simulink model "F450_model"  (R2022a)
settings: Solver=ode4  StartTime=0.0  StopTime=10  FixedStep=0.001  RelTol=1e-3
values from neighbouring files (symbols this model uses):
  motorRpm0 = [5320.31451534 5320.31451534 5320.31451534 5320.31451534]    [trim_hover.mat]
  x0 = [0 0 0 0 0 0 0 0 0 0 0 -100]    [trim_hover.mat]
undefined symbols (not defined in the file or in its folder): Cd, Cmd, d_prop, dzcg, g, Inertia, Inertia_inv, Mass, motorCr, motorJm, motorTm, motorWb, rotorCm, rotorCt
libraries: matrix_library x2, aerospace x2
settings Model: SimulationMode=accelerator  Creator=dream  LastModifiedBy=김응태
settings SolverCC: AlgebraicLoopSolver=TrustRegion
settings DataIOCC: ReturnWorkspaceOutputs=off
settings DebuggingCC: UnconnectedInputMsg=warning  UnconnectedOutputMsg=warning  UnconnectedLineMsg=warning  BusObjectLabelMismatch=error  SFMachineParentedDataDiag=warning  ArithmeticOperatorsInVariantConditions=warning
settings SFSimCC: SimUseLocalCustomCode=off  CustomCodeUndefinedFunction=UseInterfaceOnly
settings RTWCC: RTWUseLocalCustomCode=off
settings CodeAppCC: StateflowObjectComments=on

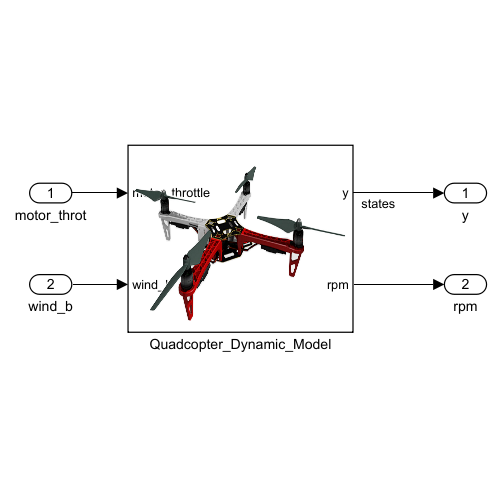
[thumbnail: Simulink's stored preview of the top-level diagram]
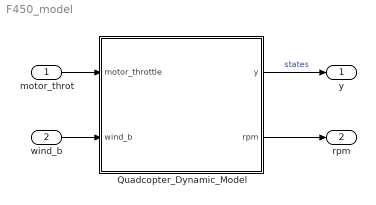
== system F450_model ==
  motor_throt : Inport
  wind_b : Inport  Port=2  PortDimensions=3
  Quadcopter_Dynamic_Model : Subsystem
      mask Display: image('F450.png'); % Use "Edit Image" on toolstrip to change.
  y : Outport
  rpm : Outport  Port=2
  wires:
  motor_throt/1 -> Quadcopter_Dynamic_Model/1(motor_throttle)
  Quadcopter_Dynamic_Model/1(y) -> y/1  "states"
  Quadcopter_Dynamic_Model/2(rpm) -> rpm/1
  wind_b/1 -> Quadcopter_Dynamic_Model/2(wind_b)

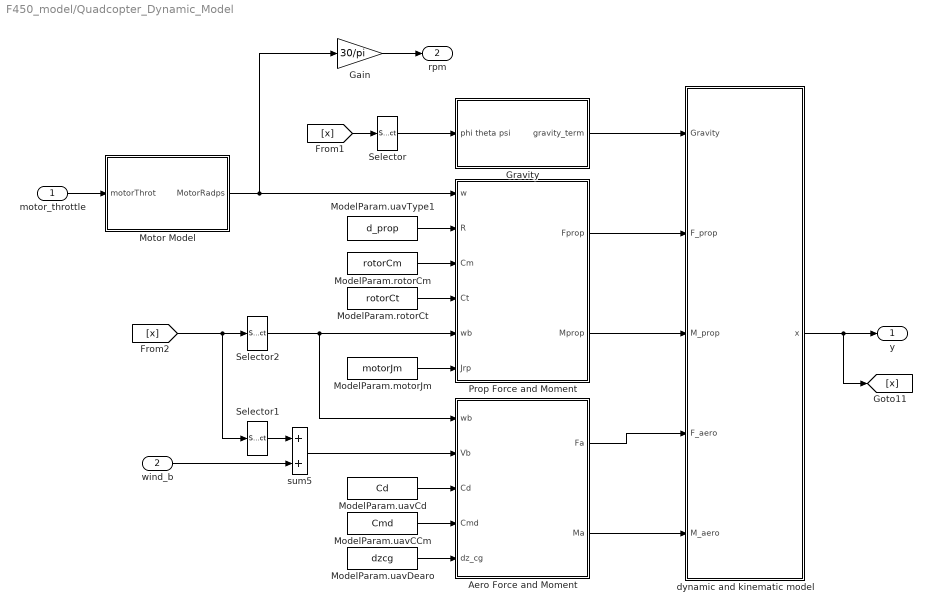
== system F450_model/Quadcopter_Dynamic_Model ==
  motor_throttle : Inport
  wind_b : Inport  Port=2
  Aero Force and Moment : MATLAB Function  TreatAsAtomicUnit=on
  Gain : Gain  Gain=30/pi
  Gravity : Subsystem
  ModelParam.motorJm : Constant  Value=motorJm
  ModelParam.rotorCm : Constant  Value=rotorCm
  ModelParam.rotorCt : Constant  Value=rotorCt
  ModelParam.uavCCm : Constant  Value=Cmd
  ModelParam.uavCd : Constant  Value=Cd
  ModelParam.uavDearo : Constant  Value=dzcg
  ModelParam.uavType1 : Constant  Value=d_prop
  Motor Model : Subsystem
  Prop Force and Moment : MATLAB Function  TreatAsAtomicUnit=on
  Selector : Selector  InputPortWidth=12  IndexOptions=Index vector (dialog)  Indices=[7 8 9]  OutputSizes=1
  Selector1 : Selector  InputPortWidth=12  IndexOptions=Index vector (dialog)  Indices=[1 2 3]  OutputSizes=1
  Selector2 : Selector  InputPortWidth=12  IndexOptions=Index vector (dialog)  Indices=[4 5 6]  OutputSizes=1
  dynamic and kinematic model : Subsystem
  sum5 : Sum  InputSameDT=on  SaturateOnIntegerOverflow=on  OutDataTypeStr=Inherit: Same as first input
  y : Outport
  rpm : Outport  Port=2
  wires:
  ModelParam.uavDearo/1 -> Aero Force and Moment/5(dz_cg)
  ModelParam.uavCCm/1 -> Aero Force and Moment/4(Cmd)
  ModelParam.uavCd/1 -> Aero Force and Moment/3(Cd)
  Aero Force and Moment/2(Ma) -> dynamic and kinematic model/5(M_aero)
  Aero Force and Moment/1(Fa) -> dynamic and kinematic model/4(F_aero)
  Prop Force and Moment/2(Mprop) -> dynamic and kinematic model/3(M_prop)
  Prop Force and Moment/1(Fprop) -> dynamic and kinematic model/2(F_prop)
  ModelParam.motorJm/1 -> Prop Force and Moment/6(Jrp)
  ModelParam.uavType1/1 -> Prop Force and Moment/2(R)
  ModelParam.rotorCt/1 -> Prop Force and Moment/4(Ct)
  ModelParam.rotorCm/1 -> Prop Force and Moment/3(Cm)
  dynamic and kinematic model/1(x) -> [x], y/1
  Gravity/1(gravity_term) -> dynamic and kinematic model/1(Gravity)
  motor_throttle/1 -> Motor Model/1(motorThrot)
  Gain/1 -> rpm/1
  Selector/1 -> Gravity/1(phi theta psi)
  [x] -> Selector/1
  [x] -> Selector2/1, Selector1/1
  Selector2/1 -> Prop Force and Moment/5(wb), Aero Force and Moment/1(wb)
  Motor Model/1(MotorRadps) -> Gain/1, Prop Force and Moment/1(w)
  wind_b/1 -> sum5/2
  Selector1/1 -> sum5/1
  sum5/1 -> Aero Force and Moment/2(Vb)

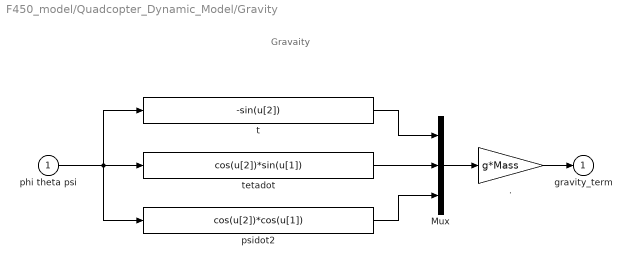
== system F450_model/Quadcopter_Dynamic_Model/Gravity ==
  note: Gravaity
  phi theta psi : Inport
  . : Gain  Gain=g*Mass  SaturateOnIntegerOverflow=on  OutDataTypeStr=Inherit: Same as input  ParamDataTypeStr=Inherit: Same as input
  Mux : Mux  Inputs=3
  psidot2 : Fcn  Expr=cos(u[2])*cos(u[1])
  t : Fcn  Expr=-sin(u[2])
  tetadot : Fcn  Expr=cos(u[2])*sin(u[1])
  gravity_term : Outport  InitialOutput=0  VectorParamsAs1DForOutWhenUnconnected=off
  wires:
  t/1 -> Mux/1
  psidot2/1 -> Mux/3
  tetadot/1 -> Mux/2
  Mux/1 -> ./1
  phi theta psi/1 -> tetadot/1, t/1, psidot2/1
  ./1 -> gravity_term/1

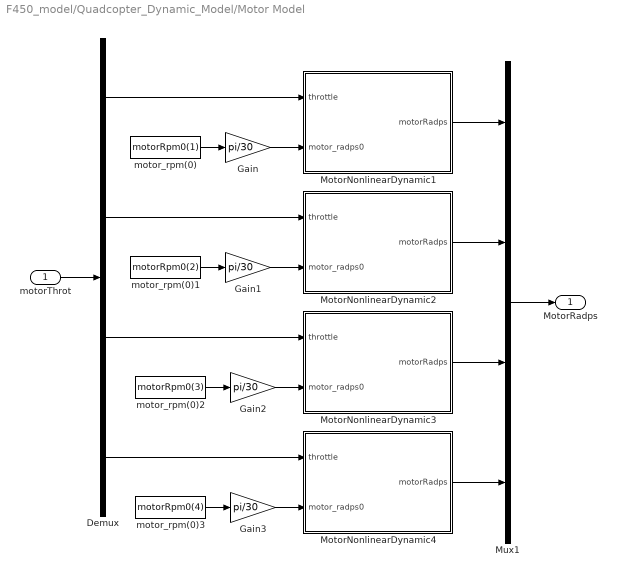
== system F450_model/Quadcopter_Dynamic_Model/Motor Model ==
  motorThrot : Inport
  Demux : Demux
  Gain{,1..3} (4 alike) : Gain  Gain=pi/30
  MotorNonlinearDynamic1 : Subsystem  TreatAsAtomicUnit=on
  MotorNonlinearDynamic2 : Subsystem  TreatAsAtomicUnit=on
  MotorNonlinearDynamic3 : Subsystem  TreatAsAtomicUnit=on
  MotorNonlinearDynamic4 : Subsystem  TreatAsAtomicUnit=on
  Mux1 : Mux
  motor_rpm(0) : Constant  Value=motorRpm0(1)
  motor_rpm(0)1 : Constant  Value=motorRpm0(2)
  motor_rpm(0)2 : Constant  Value=motorRpm0(3)
  motor_rpm(0)3 : Constant  Value=motorRpm0(4)
  MotorRadps : Outport  VectorParamsAs1DForOutWhenUnconnected=off
  wires:
  motorThrot/1 -> Demux/1
  Demux/4 -> MotorNonlinearDynamic4/1(throttle)
  motor_rpm(0)/1 -> Gain/1
  MotorNonlinearDynamic3/1(motorRadps) -> Mux1/3
  MotorNonlinearDynamic2/1(motorRadps) -> Mux1/2
  Mux1/1 -> MotorRadps/1
  Demux/2 -> MotorNonlinearDynamic2/1(throttle)
  Demux/3 -> MotorNonlinearDynamic3/1(throttle)
  Demux/1 -> MotorNonlinearDynamic1/1(throttle)
  MotorNonlinearDynamic4/1(motorRadps) -> Mux1/4
  MotorNonlinearDynamic1/1(motorRadps) -> Mux1/1
  Gain/1 -> MotorNonlinearDynamic1/2(motor_radps0)
  motor_rpm(0)1/1 -> Gain1/1
  Gain1/1 -> MotorNonlinearDynamic2/2(motor_radps0)
  motor_rpm(0)2/1 -> Gain2/1
  Gain2/1 -> MotorNonlinearDynamic3/2(motor_radps0)
  motor_rpm(0)3/1 -> Gain3/1
  Gain3/1 -> MotorNonlinearDynamic4/2(motor_radps0)

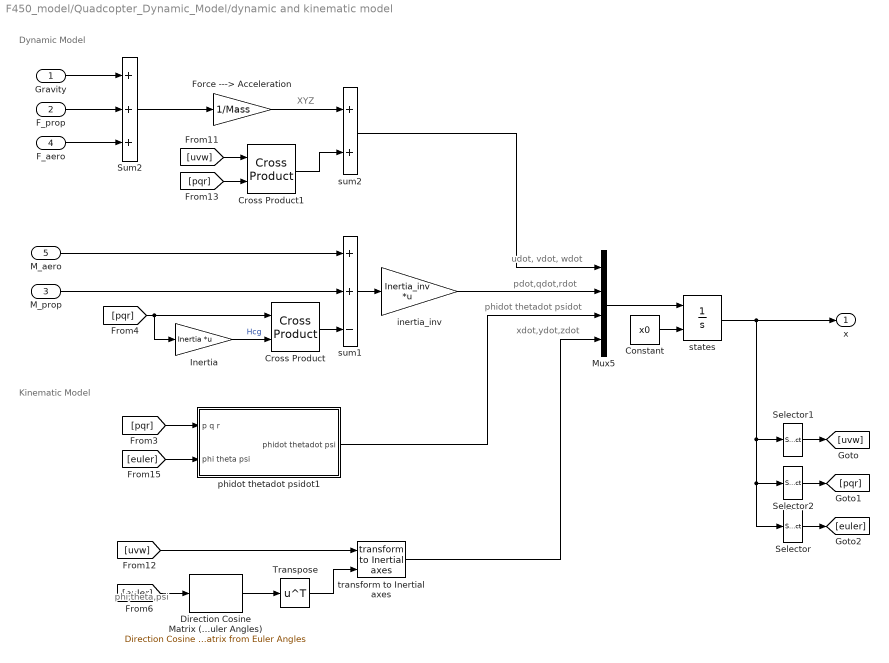
== system F450_model/Quadcopter_Dynamic_Model/dynamic and kinematic model ==
  note: Kinematic Model
  note: phi,theta,psi
  note: udot, vdot, wdot
  note: pdot,qdot,rdot
  note: phidot thetadot psidot
  note: xdot,ydot,zdot
  note: XYZ
  note: Dynamic Model
  Gravity : Inport
  F_prop : Inport  Port=2
  M_prop : Inport  Port=3
  F_aero : Inport  Port=4
  M_aero : Inport  Port=5
  Constant : Constant  Value=x0
  Cross Product : matrix_library/Cross Product
      settings: SourceProductBaseCode=SL
  Cross Product1 : matrix_library/Cross Product
      settings: SourceProductBaseCode=SL
  Direction Cosine Matrix (Euler Angles) : aerospace/Axes Transformations/Direction Cosine Matrix from Euler Angles
      settings: SourceProductBaseCode=SL
  Force ---> Acceleration : Gain  Gain=1/Mass  SaturateOnIntegerOverflow=on  OutDataTypeStr=Inherit: Same as input  ParamDataTypeStr=Inherit: Same as input
  Inertia : Gain  Gain=Inertia  Multiplication=Matrix(K*u)
  Mux5 : Mux
  Selector : Selector  InputPortWidth=12  IndexOptions=Index vector (dialog)  Indices=[7 8 9]  OutputSizes=1
  Selector1 : Selector  InputPortWidth=12  IndexOptions=Index vector (dialog)  Indices=[1 2 3]  OutputSizes=1
  Selector2 : Selector  InputPortWidth=12  IndexOptions=Index vector (dialog)  Indices=[4 5 6]  OutputSizes=1
  Sum2 : Sum  Inputs=+++  InputSameDT=on  SaturateOnIntegerOverflow=on  OutDataTypeStr=Inherit: Same as first input
  Transpose : Math  Operator=transpose  SignedPower=on
  inertia_inv : Gain  Gain=Inertia_inv  Multiplication=Matrix(K*u)
  phidot thetadot psidot1 : Subsystem
  states : Integrator  InitialConditionSource=external  InitialCondition=x0
  sum1 : Sum  Inputs=++-  InputSameDT=on  SaturateOnIntegerOverflow=on  OutDataTypeStr=Inherit: Same as first input
  sum2 : Sum  InputSameDT=on  SaturateOnIntegerOverflow=on  OutDataTypeStr=Inherit: Same as first input
  "transform to Inertial axes " : aerospace/6DoF/Euler Angles/transform to Inertial axes   SystemSampleTime=-1  VariantActivationTime=update diagram  Latency=0  AutoFrameSizeCalculation=off
      settings: SourceProductBaseCode=SL
  x : Outport  VectorParamsAs1DForOutWhenUnconnected=off
  wires:
  M_prop/1 -> sum1/2
  Cross Product/1 -> sum1/3
  M_aero/1 -> sum1/1
  F_aero/1 -> Sum2/3
  F_prop/1 -> Sum2/2
  Gravity/1 -> Sum2/1
  Sum2/1 -> Force ---> Acceleration/1
  Force ---> Acceleration/1 -> sum2/1
  Cross Product1/1 -> sum2/2
  sum1/1 -> inertia_inv/1
  Inertia/1 -> Cross Product/2  "Hcg"
  phidot thetadot psidot1/1(phidot thetadot psi) -> Mux5/3
  Direction Cosine Matrix (Euler Angles)/1 -> Transpose/1
  sum2/1 -> Mux5/1
  Transpose/1 -> "transform to Inertial axes "/2
  inertia_inv/1 -> Mux5/2
  Mux5/1 -> states/1
  [pqr] -> Inertia/1, Cross Product/1
  [uvw] -> Cross Product1/1
  [uvw] -> "transform to Inertial axes "/1
  [pqr] -> Cross Product1/2
  [euler] -> phidot thetadot psidot1/2(phi theta psi)
  "transform to Inertial axes "/1 -> Mux5/4
  [pqr] -> phidot thetadot psidot1/1(p q r)
  [euler] -> Direction Cosine Matrix (Euler Angles)/1
  Selector2/1 -> [pqr]
  Selector1/1 -> [uvw]
  Constant/1 -> states/2
  Selector/1 -> [euler]
  states/1 -> x/1, Selector1/1, Selector/1, Selector2/1

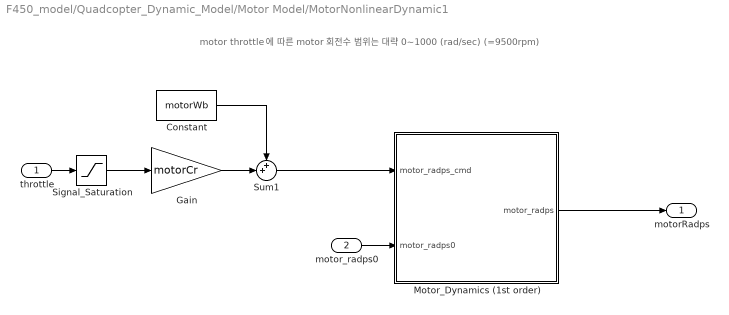
== system F450_model/Quadcopter_Dynamic_Model/Motor Model/MotorNonlinearDynamic1 ==
  note: motor throttle 에 따른 motor 회전수 범위는 대략 0~1000 (rad/sec) (=9500rpm)
  throttle : Inport
  motor_radps0 : Inport  Port=2
  Constant : Constant  Value=motorWb
  Gain : Gain  Gain=motorCr
  Motor_Dynamics (1st order) : Subsystem  TreatAsAtomicUnit=on
  Signal_Saturation : Saturate  UpperLimit=0.95  LowerLimit=0
      settings: AttributesFormatString=%<LowerLimit>~%<UpperLimit>
  Sum1 : Sum  Inputs=++|
  motorRadps : Outport  VectorParamsAs1DForOutWhenUnconnected=off
  wires:
  Motor_Dynamics (1st order)/1(motor_radps) -> motorRadps/1
  motor_radps0/1 -> Motor_Dynamics (1st order)/2(motor_radps0)
  Constant/1 -> Sum1/1
  Gain/1 -> Sum1/2
  Signal_Saturation/1 -> Gain/1
  Sum1/1 -> Motor_Dynamics (1st order)/1(motor_radps_cmd)
  throttle/1 -> Signal_Saturation/1

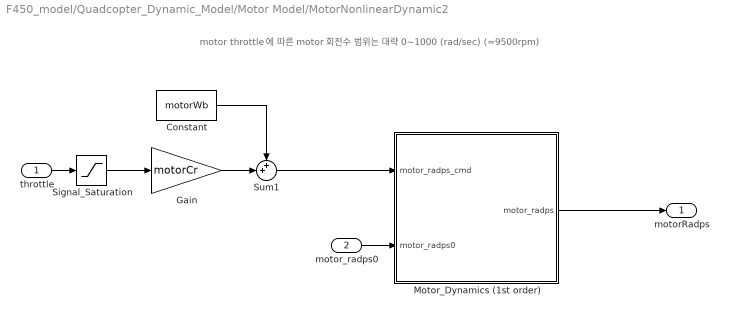
== system F450_model/Quadcopter_Dynamic_Model/Motor Model/MotorNonlinearDynamic2 ==
  note: motor throttle 에 따른 motor 회전수 범위는 대략 0~1000 (rad/sec) (=9500rpm)
  throttle : Inport
  motor_radps0 : Inport  Port=2
  Constant : Constant  Value=motorWb
  Gain : Gain  Gain=motorCr
  Motor_Dynamics (1st order) : Subsystem  TreatAsAtomicUnit=on
  Signal_Saturation : Saturate  UpperLimit=0.95  LowerLimit=0
      settings: AttributesFormatString=%<LowerLimit>~%<UpperLimit>
  Sum1 : Sum  Inputs=++|
  motorRadps : Outport  VectorParamsAs1DForOutWhenUnconnected=off
  wires:
  throttle/1 -> Signal_Saturation/1
  Sum1/1 -> Motor_Dynamics (1st order)/1(motor_radps_cmd)
  Signal_Saturation/1 -> Gain/1
  Gain/1 -> Sum1/2
  Constant/1 -> Sum1/1
  motor_radps0/1 -> Motor_Dynamics (1st order)/2(motor_radps0)
  Motor_Dynamics (1st order)/1(motor_radps) -> motorRadps/1

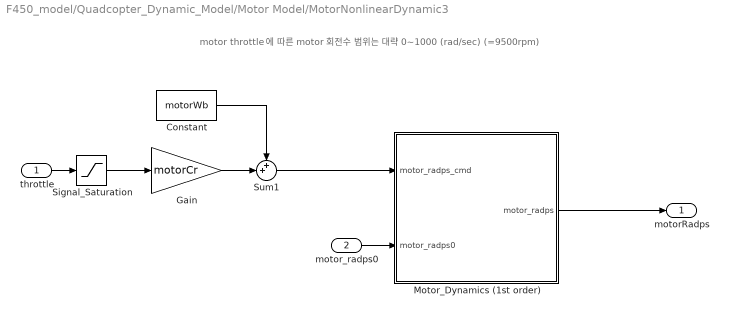
== system F450_model/Quadcopter_Dynamic_Model/Motor Model/MotorNonlinearDynamic3 ==
  note: motor throttle 에 따른 motor 회전수 범위는 대략 0~1000 (rad/sec) (=9500rpm)
  throttle : Inport
  motor_radps0 : Inport  Port=2
  Constant : Constant  Value=motorWb
  Gain : Gain  Gain=motorCr
  Motor_Dynamics (1st order) : Subsystem  TreatAsAtomicUnit=on
  Signal_Saturation : Saturate  UpperLimit=0.95  LowerLimit=0
      settings: AttributesFormatString=%<LowerLimit>~%<UpperLimit>
  Sum1 : Sum  Inputs=++|
  motorRadps : Outport  VectorParamsAs1DForOutWhenUnconnected=off
  wires:
  Motor_Dynamics (1st order)/1(motor_radps) -> motorRadps/1
  motor_radps0/1 -> Motor_Dynamics (1st order)/2(motor_radps0)
  Constant/1 -> Sum1/1
  Gain/1 -> Sum1/2
  Signal_Saturation/1 -> Gain/1
  Sum1/1 -> Motor_Dynamics (1st order)/1(motor_radps_cmd)
  throttle/1 -> Signal_Saturation/1

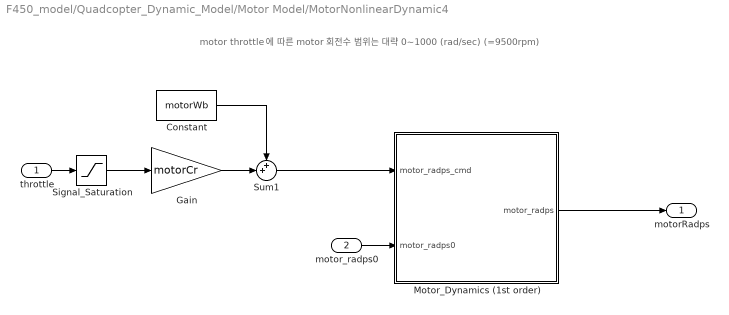
== system F450_model/Quadcopter_Dynamic_Model/Motor Model/MotorNonlinearDynamic4 ==
  note: motor throttle 에 따른 motor 회전수 범위는 대략 0~1000 (rad/sec) (=9500rpm)
  throttle : Inport
  motor_radps0 : Inport  Port=2
  Constant : Constant  Value=motorWb
  Gain : Gain  Gain=motorCr
  Motor_Dynamics (1st order) : Subsystem  TreatAsAtomicUnit=on
  Signal_Saturation : Saturate  UpperLimit=0.95  LowerLimit=0
      settings: AttributesFormatString=%<LowerLimit>~%<UpperLimit>
  Sum1 : Sum  Inputs=++|
  motorRadps : Outport  VectorParamsAs1DForOutWhenUnconnected=off
  wires:
  throttle/1 -> Signal_Saturation/1
  Sum1/1 -> Motor_Dynamics (1st order)/1(motor_radps_cmd)
  Signal_Saturation/1 -> Gain/1
  Gain/1 -> Sum1/2
  Constant/1 -> Sum1/1
  motor_radps0/1 -> Motor_Dynamics (1st order)/2(motor_radps0)
  Motor_Dynamics (1st order)/1(motor_radps) -> motorRadps/1

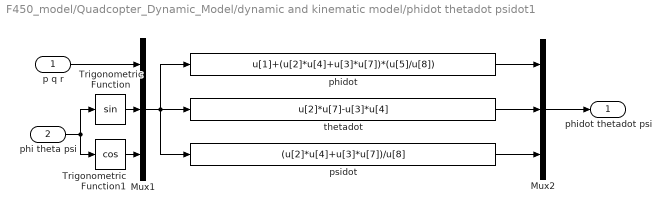
== system F450_model/Quadcopter_Dynamic_Model/dynamic and kinematic model/phidot thetadot psidot1 ==
  p q r : Inport
  phi theta psi : Inport  Port=2
  Mux1 : Mux  Inputs=[3 3 3]
  Mux2 : Mux  Inputs=3
  Trigonometric Function : Trigonometry
  Trigonometric Function1 : Trigonometry  Operator=cos
  phidot : Fcn  Expr=u[1]+(u[2]*u[4]+u[3]*u[7])*(u[5]/u[8])
  psidot : Fcn  Expr=(u[2]*u[4]+u[3]*u[7])/u[8]
  thetadot : Fcn  Expr=u[2]*u[7]-u[3]*u[4]
  phidot thetadot psi : Outport  InitialOutput=0  VectorParamsAs1DForOutWhenUnconnected=off
  wires:
  Trigonometric Function1/1 -> Mux1/3
  Trigonometric Function/1 -> Mux1/2
  Mux2/1 -> phidot thetadot psi/1
  phidot/1 -> Mux2/1
  thetadot/1 -> Mux2/2
  psidot/1 -> Mux2/3
  phi theta psi/1 -> Trigonometric Function1/1, Trigonometric Function/1
  p q r/1 -> Mux1/1
  Mux1/1 -> thetadot/1, phidot/1, psidot/1

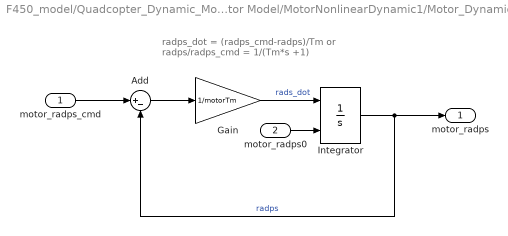
== system F450_model/Quadcopter_Dynamic_Model/Motor Model/MotorNonlinearDynamic1/Motor_Dynamics (1st order) ==
  note: radps_dot = (radps_cmd-radps)/Tm
      | or
      | radps/radps_cmd = 1/(Tm*s +1)
  motor_radps_cmd : Inport
  motor_radps0 : Inport  Port=2
  Add : Sum  Inputs=|+-
  Gain : Gain  Gain=1/motorTm
  Integrator : Integrator  InitialConditionSource=external
  motor_radps : Outport  VectorParamsAs1DForOutWhenUnconnected=off
  wires:
  Add/1 -> Gain/1
  motor_radps0/1 -> Integrator/2
  motor_radps_cmd/1 -> Add/1
  Gain/1 -> Integrator/1  "rads_dot"
  Integrator/1 -> Add/2, motor_radps/1  "radps"

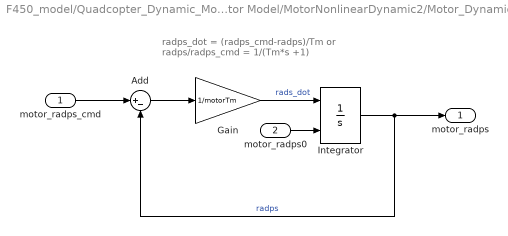
== system F450_model/Quadcopter_Dynamic_Model/Motor Model/MotorNonlinearDynamic2/Motor_Dynamics (1st order) ==
  note: radps_dot = (radps_cmd-radps)/Tm
      | or
      | radps/radps_cmd = 1/(Tm*s +1)
  motor_radps_cmd : Inport
  motor_radps0 : Inport  Port=2
  Add : Sum  Inputs=|+-
  Gain : Gain  Gain=1/motorTm
  Integrator : Integrator  InitialConditionSource=external
  motor_radps : Outport  VectorParamsAs1DForOutWhenUnconnected=off
  wires:
  Integrator/1 -> motor_radps/1, Add/2  "radps"
  Gain/1 -> Integrator/1  "rads_dot"
  motor_radps_cmd/1 -> Add/1
  motor_radps0/1 -> Integrator/2
  Add/1 -> Gain/1

== system F450_model/Quadcopter_Dynamic_Model/Motor Model/MotorNonlinearDynamic3/Motor_Dynamics (1st order) ==
  note: radps_dot = (radps_cmd-radps)/Tm
      | or
      | radps/radps_cmd = 1/(Tm*s +1)
  motor_radps_cmd : Inport
  motor_radps0 : Inport  Port=2
  Add : Sum  Inputs=|+-
  Gain : Gain  Gain=1/motorTm
  Integrator : Integrator  InitialConditionSource=external
  motor_radps : Outport  VectorParamsAs1DForOutWhenUnconnected=off
  wires:
  Add/1 -> Gain/1
  motor_radps0/1 -> Integrator/2
  motor_radps_cmd/1 -> Add/1
  Gain/1 -> Integrator/1  "rads_dot"
  Integrator/1 -> Add/2, motor_radps/1  "radps"

== system F450_model/Quadcopter_Dynamic_Model/Motor Model/MotorNonlinearDynamic4/Motor_Dynamics (1st order) ==
  note: radps_dot = (radps_cmd-radps)/Tm
      | or
      | radps/radps_cmd = 1/(Tm*s +1)
  motor_radps_cmd : Inport
  motor_radps0 : Inport  Port=2
  Add : Sum  Inputs=|+-
  Gain : Gain  Gain=1/motorTm
  Integrator : Integrator  InitialConditionSource=external
  motor_radps : Outport  VectorParamsAs1DForOutWhenUnconnected=off
  wires:
  Integrator/1 -> motor_radps/1, Add/2  "radps"
  Gain/1 -> Integrator/1  "rads_dot"
  motor_radps_cmd/1 -> Add/1
  motor_radps0/1 -> Integrator/2
  Add/1 -> Gain/1

== matlab function F450_model/Quadcopter_Dynamic_Model/Aero Force and Moment ==
  data: Fa output; Ma output; wb input; Vb input; Cd input; Cmd input; dz_cg input
function [Fa,Ma] = fcn(wb,Vb,Cd,Cmd,dz_cg)

 Fa = -Cd*Vb.*abs(Vb);         % Careful for the definition of Cd

 Md = -Cmd.*wb.*abs(wb);       % aerodynamic damping moment
  
 Mfd= [Fa(2)*dz_cg
      -Fa(1)*dz_cg
       0];

 Ma = Mfd + Md;
 
end

== matlab function F450_model/Quadcopter_Dynamic_Model/Prop Force and Moment ==
  data: w input; R input; Cm input; Ct input; Fprop output; Mprop output; wb input; Jrp input
function [Fprop, Mprop] = fcn(w, R, Cm, Ct, wb, Jrp)

 %  Obtain the force and torque acting on the body. 
 %  The airframe of the quadrotor is as follows:
 %  3↓   1↑
 %    \ /
 %    / \
 %  2↑   4↓
 %  ↑ stands for counterclockwise and ↓stands for clockwise.
 
 % Input：
 %  w: motor speed，unit：rad/s
 %  R: body radius(m)
 %  Cm: torque coefficient
 %  Ct: thrust coefficient
 %  wb: angular velocity in the body coordinate system
 %  Jrp:  moment of inertia of motor rotor + propeller

 % Output:
 %  Fprop: force vector from prop
 %  Mprop: aerodynamic damping moment + gyro moment

 
 F_prop = Ct*(w.^2);      % Force from each prop
 M_prop = Cm*(w.^2);      % Torque magnitude from each prop

 Fprop = [0; 0; -sum(F_prop)];

 d=sin(pi/4)*R;
 Mp= [ d*F_prop'*[-1;  1;  1; -1]
       d*F_prop'*[ 1; -1;  1; -1]
         M_prop'*[ 1;  1; -1; -1] ];

% gyro moment
 M_gyro   = [Jrp*wb(2)*( w(1) + w(2) - w(3) - w(4));  
             Jrp*wb(1)*(-w(1) - w(2) + w(3) + w(4));
             0];

 Mprop = Mp + M_gyro;

end
